simulink model "Model1"  (R2020a)
settings: Solver=VariableStepAuto  StartTime=0.0  StopTime=1600 * SimPars.SampleTime  RelTol=1e-3
undefined symbols (not defined in the file or in its folder): pskmod, SimPars
libraries: commutil2 x4, commdigbbndpm3 x3, dspsigops x2, commsequence2 x2, commsync2 x2, commfilt2 x2, commrflib2 x1, commsink2 x1, commrfcorlib x1, dspstat3 x1, commrandsrc3 x1, dspmathops x1
settings Model: Creator=esha_  LastModifiedBy=esha_

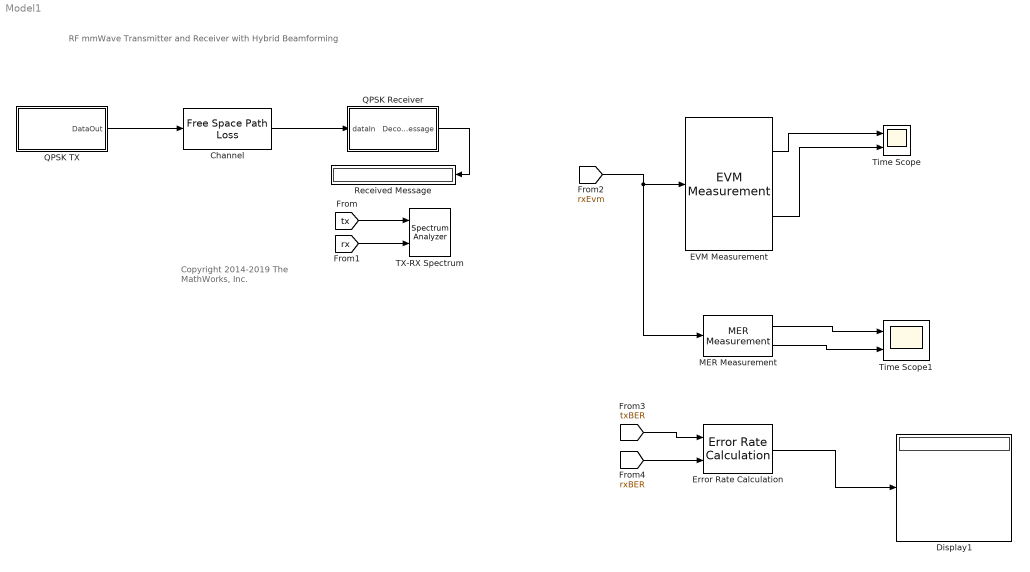
== system Model1 ==
  note: RF mmWave Transmitter and Receiver with Hybrid Beamforming
  note: Copyright 2014-2019 The MathWorks, Inc.
  Channel : commrflib2/Free Space Path Loss  mode=Decibels  dB=5  d=0.100  fc=1920
      settings: SourceProductBaseCode=CM
  Display1 : Display
  EVM Measurement : commutil2/EVM Measurement  Normalization=Average reference signal power  AverageConstellationPower=1  PeakConstellationPower=1  ReferenceSignalSource=Estimated from reference constellation  ReferenceConstellation=pskmod((0:3),4,pi/4)  MeasurementIntervalSource=Input length  MeasurementInterval=100  AveragingDimensions=1  MaximumEVMOutputPort=on  XPercentileEVMOutputPort=off  XPercentileValue=95  SymbolCountOutputPort=on  SimulateUsing=Interpreted execution
      settings: SourceProductBaseCode=CM
  Error Rate Calculation : commsink2/Error Rate Calculation  N=0  st_delay=0  cp_mode=Entire frame  subframe=[]  PMode=Port  WsName=ErrorVec  RsMode2=off  stop=off  numErr=100  maxBits=1e6
  MER Measurement : commutil2/MER Measurement  ReferenceSignalSource=Estimated from reference constellation  ReferenceConstellation=pskmod((0:3),4,pi/4)  MeasurementIntervalSource=Input length  MeasurementInterval=100  AveragingDimensions=1  MinimumMEROutputPort=on  XPercentileMEROutputPort=off  XPercentileValue=95  SymbolCountOutputPort=off  SimulateUsing=Interpreted execution
      settings: SourceProductBaseCode=CM
  QPSK Receiver : Subsystem
      mask Display: disp('QPSK \n Receiver');
  QPSK TX : Subsystem  mask{Power=-10}
      mask prompts: Power "Power (dBFS)"
      mask Display: disp('QPSK \n Transmitter')
  Received Message : Display
  TX-RX Spectrum : SpectrumAnalyzer  NumInputPorts=2
  Time Scope : Scope  NumInputPorts=2
      settings: Description=EVM
  Time Scope1 : Scope  NumInputPorts=2
      settings: Description=SNR
  wires:
  [rx] -> TX-RX Spectrum/2
  QPSK Receiver/1(Decoded Message) -> Received Message/1
  [tx] -> TX-RX Spectrum/1
  QPSK TX/1(DataOut) -> Channel/1
  Channel/1 -> QPSK Receiver/1(dataIn)
  EVM Measurement/1 -> Time Scope/1
  EVM Measurement/2 -> Time Scope/2
  [rxEvm] -> MER Measurement/1, EVM Measurement/1
  MER Measurement/1 -> Time Scope1/1
  MER Measurement/2 -> Time Scope1/2
  Error Rate Calculation/1 -> Display1/1
  [txBER] -> Error Rate Calculation/1
  [rxBER] -> Error Rate Calculation/2

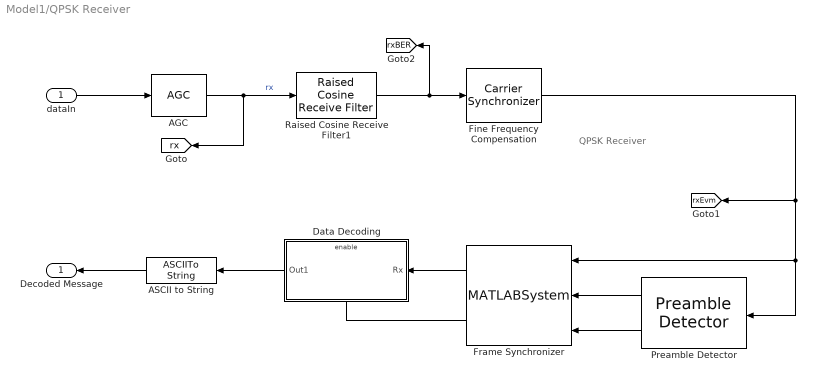
== system Model1/QPSK Receiver ==
  note: QPSK Receiver
  dataIn : Inport
  AGC : commrfcorlib/AGC  LegacyMode=off  DetectorMethod=Rectifier  LoopMethod=Linear  UpdatePeriod=100  StepSize=0.1  AdaptationStepSize=0.01  DesiredOutputPower=1  AveragingLength=200  MaximumGain=30  MaxPowerGain=60  GainOutputPort=off  InputPowerOutputPort=off  SimulateUsing=Code generation
  ASCII to String : ASCIIToString
  Data Decoding : Subsystem
      mask Display: disp('Data Decoding');
  Fine Frequency Compensation : commsync2/Carrier Synchronizer  Modulation=QPSK  ModulationPhaseOffset=Auto  CustomPhaseOffset=0  SamplesPerSymbol=1  DampingFactor=1/sqrt(2)  NormalizedLoopBandwidth=0.005  EstimatedPhaseErrorOutputPort=off  SimulateUsing=Code generation
  Frame Synchronizer : MATLABSystem  System=comm.internal.examples.FrameSynchronizer  Input=Symbol  OutputFrameLength=SimPars.NumSymsPerFrame  PreambleLength=SimPars.BarkerLength  SimulateUsing=Code generation
      mask Type: comm.internal.examples.FrameSynchronizer
      mask Display:
      | disp(['Frame' char(10) 'Synchronizer']);
      | port_label('input',1,'u');
      | port_label('input',2,'idx');
      | port_label('input',3,'dtMt');
      | port_label('output',1,'Frame');
      | port_label('output',2,'Valid');
  Preamble Detector : commsync2/Preamble Detector  Input=Symbol  Preamble=sqrt(2)/2 * (-1-1i) *SimPars.BarkerCode  Threshold=10  DetectionMetricOutput=on  Detections=All  SimulateUsing=Code generation
      settings: SourceProductBaseCode=CM
  Raised Cosine Receive Filter1 : commfilt2/Raised Cosine Receive Filter  filtType=Square root  R=SimPars.RolloffFactor  filtSpan=SimPars.RCFilterSpan  N=SimPars.SamplesPerSymbol  downFactor=SimPars.RxRCFilterDecimation  downOffset=0  filterGain=1  InputProcessing=Columns as channels (frame based)  RateOptions=Enforce single-rate processing  framing=Mute  checkCoeff=off  variableName=rcRxFilt1  currentFiltSpan=10  D=5  inputOffset=0  sampMode=Mute  saveAsFlag=0  rateMode=Downsampling  checkGain=Normalized  launchFVT=on  roundingMode=Floor  overflowMode=off  coeffDataTypeStr=Inherit: Same word length as input  coeffMin=[]  coeffMax=[]  coeffLastDataTypeStr=Inherit: Same word length as input  accumDataTypeStr=Inherit: Same as product output  accumLastDataTypeStr=Inherit: Same as product output  outputDataTypeStr=Inherit: Same as accumulator  outputMin=[]  outputMax=[]  outputLastDataTypeStr=Inherit: Same as accumulator
  Decoded Message : Outport  VectorParamsAs1DForOutWhenUnconnected=off
  tag scope: rx=global, rxBER=global, rxEvm=global
  wires:
  ASCII to String/1 -> Decoded Message/1
  Data Decoding/1(Out1) -> ASCII to String/1
  AGC/1 -> Raised Cosine Receive Filter1/1, [rx]  "rx"
  Preamble Detector/1 -> Frame Synchronizer/2
  Frame Synchronizer/2 -> Data Decoding/Enable
  Frame Synchronizer/1 -> Data Decoding/1(Rx)
  Preamble Detector/2 -> Frame Synchronizer/3
  Fine Frequency Compensation/1 -> [rxEvm], Frame Synchronizer/1, Preamble Detector/1
  dataIn/1 -> AGC/1
  Raised Cosine Receive Filter1/1 -> [rxBER], Fine Frequency Compensation/1

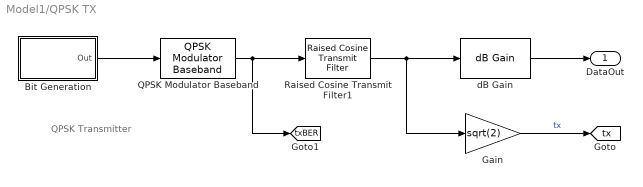
== system Model1/QPSK TX ==
  note: QPSK Transmitter
  Bit Generation : Subsystem
      mask Display: disp('Bits Generation')
  Gain : Gain  Gain=sqrt(2)
  QPSK Modulator Baseband : commdigbbndpm3/QPSK Modulator Baseband  InType=Bit  Enc=Gray  Ph=pi/4  outDtype=double  outWordLen=16  outUDDataType=sfix(16)  outFracLenMode=Best precision  outFracLen=15  outDataTypeStr=double  outLastDataTypeStr=double
  Raised Cosine Transmit Filter1 : commfilt2/Raised Cosine Transmit Filter  filtType=Square root  R=SimPars.RolloffFactor  filtSpan=SimPars.RCFilterSpan  N=SimPars.SamplesPerSymbol  filterGain=1  InputProcessing=Columns as channels (frame based)  RateOptions=Enforce single-rate processing  framing=Mute  checkCoeff=off  variableName=rcTxFilt1  checkGain=Normalized  sampMode=Mute  saveAsFlag=0  currentFiltSpan=10  D=5  launchFVT=on  roundingMode=Floor  overflowMode=off  coeffDataTypeStr=Inherit: Same word length as input  coeffMin=[]  coeffMax=[]  coeffLastDataTypeStr=Inherit: Same word length as input  outputDataTypeStr=Inherit: Same as accumulator  outputMin=[]  outputMax=[]  outputLastDataTypeStr=Inherit: Same as accumulator
  dB Gain : dspmathops/dB Gain  dB=Power-30+3  intype=Amplitude
      settings: SourceProductBaseCode=DS
  DataOut : Outport  VectorParamsAs1DForOutWhenUnconnected=off
  tag scope: tx=global, txBER=global
  wires:
  dB Gain/1 -> DataOut/1
  Bit Generation/1(Out) -> QPSK Modulator Baseband/1
  QPSK Modulator Baseband/1 -> [txBER], Raised Cosine Transmit Filter1/1
  Raised Cosine Transmit Filter1/1 -> Gain/1, dB Gain/1
  Gain/1 -> [tx]  "tx"

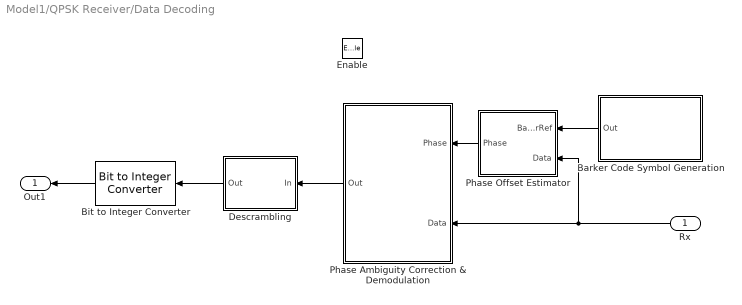
== system Model1/QPSK Receiver/Data Decoding ==
  Rx : Inport
  Enable : EnablePort
  "Barker Code Symbol Generation " : Subsystem
      mask Display: disp('Barker Code\nSymbol Generation')
  Bit to Integer Converter : commutil2/Bit to Integer Converter  nbits=7  bitOrder=MSB first  signedOutputValues=Unsigned  outDtype=Inherit via internal rule  outDtypeSigned=Inherit via internal rule
  Descrambling : Subsystem
      mask Display: disp('Descrambling');
  Phase Ambiguity Correction & Demodulation : Subsystem
      mask Display: disp('Phase Ambiguity\nCorrection\n& Demodulation');
  Phase Offset Estimator : Subsystem
  Out1 : Outport  VectorParamsAs1DForOutWhenUnconnected=off
  wires:
  "Barker Code Symbol Generation "/1(Out) -> Phase Offset Estimator/1(BarkerRef)
  Phase Offset Estimator/1(Phase) -> Phase Ambiguity Correction & Demodulation/1(Phase)
  Rx/1 -> Phase Offset Estimator/2(Data), Phase Ambiguity Correction & Demodulation/2(Data)
  Descrambling/1(Out) -> Bit to Integer Converter/1
  Phase Ambiguity Correction & Demodulation/1(Out) -> Descrambling/1(In)
  Bit to Integer Converter/1 -> Out1/1

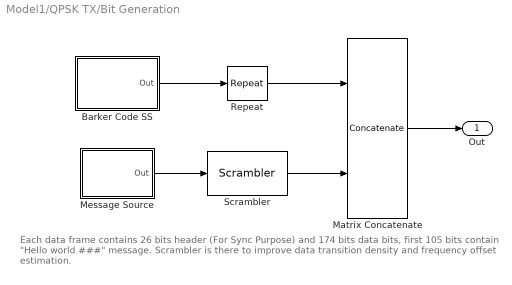
== system Model1/QPSK TX/Bit Generation ==
  note: Each data frame contains 26 bits header (For Sync Purpose) and 174 bits data bits, first 105 bits contain "Hello world ###" message. Scrambler is there to improve data transition density and frequency offset estimation.
  Barker Code SS : Subsystem
      mask Display: disp('Unipolar\nBarker Code')
  Matrix Concatenate : Concatenate  Mode=Multidimensional array
  Message Source : Subsystem
      mask Display: disp('Message\nSource')
  Repeat : dspsigops/Repeat  N=2  InputProcessing=Columns as channels (frame based)  RateOptions=Enforce single-rate processing  ic=0  mode=Unused parameter value
  Scrambler : commsequence2/Scrambler  M=2  poly=[1 1 1 0 1]  iniStaSource=Dialog Parameter  ini_sta=[0 0 0 0]  resetViaPort=off
      settings: SourceProductBaseCode=CM
  Out : Outport  VectorParamsAs1DForOutWhenUnconnected=off
  wires:
  Barker Code SS/1(Out) -> Repeat/1
  Matrix Concatenate/1 -> Out/1
  Message Source/1(Out) -> Scrambler/1
  Repeat/1 -> Matrix Concatenate/1
  Scrambler/1 -> Matrix Concatenate/2

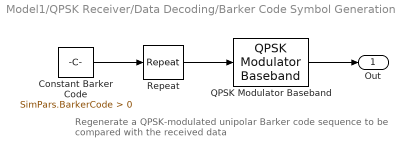
== system Model1/QPSK Receiver/Data Decoding/Barker Code Symbol Generation  ==
  note: Regenerate a QPSK-modulated unipolar Barker code sequence
      | to be compared with the received data
  Constant Barker Code : Constant  Value=SimPars.BarkerCode > 0  VectorParams1D=off  OutDataTypeStr=double
  QPSK Modulator Baseband : commdigbbndpm3/QPSK Modulator Baseband  InType=Bit  Enc=Gray  Ph=pi/4  outDtype=double  outWordLen=16  outUDDataType=sfix(16)  outFracLenMode=Best precision  outFracLen=15  outDataTypeStr=double  outLastDataTypeStr=double
  Repeat : dspsigops/Repeat  N=2  InputProcessing=Columns as channels (frame based)  RateOptions=Enforce single-rate processing  ic=0  mode=Unused parameter value
  Out : Outport  VectorParamsAs1DForOutWhenUnconnected=off
  wires:
  Constant Barker Code/1 -> Repeat/1
  Repeat/1 -> QPSK Modulator Baseband/1
  QPSK Modulator Baseband/1 -> Out/1

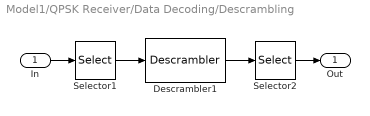
== system Model1/QPSK Receiver/Data Decoding/Descrambling ==
  In : Inport
  Descrambler1 : commsequence2/Descrambler  M=2  poly=[1 1 1 0 1]  iniStaSource=Dialog Parameter  ini_sta=[0 0 0 0]  resetViaPort=off
      settings: SourceProductBaseCode=CM
  Selector1 : Selector  IndexOptions=Index vector (dialog)  Indices=[2*SimPars.BarkerLength+1:SimPars.NumBitsPerFrame]  OutputSizes=1
  Selector2 : Selector  IndexOptions=Index vector (dialog)  Indices=[1:SimPars.NumMsgBits]  OutputSizes=1
  Out : Outport  VectorParamsAs1DForOutWhenUnconnected=off
  wires:
  In/1 -> Selector1/1
  Selector1/1 -> Descrambler1/1
  Descrambler1/1 -> Selector2/1
  Selector2/1 -> Out/1

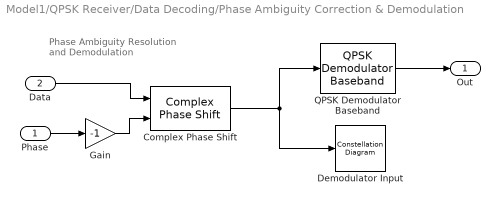
== system Model1/QPSK Receiver/Data Decoding/Phase Ambiguity Correction & Demodulation ==
  note: Phase Ambiguity Resolution
      | and Demodulation
  Phase : Inport
  Data : Inport  Port=2
  Complex Phase Shift : commutil2/Complex Phase Shift
      settings: SourceProductBaseCode=CM
  Demodulator Input : ConstellationDiagram
  Gain : Gain  Gain=-1  OutDataTypeStr=Inherit: Same as input
  QPSK Demodulator Baseband : commdigbbndpm3/QPSK Demodulator Baseband  OutType=Bit  DecType=Hard decision  VarSource=Dialog  Variance=1  Dec=Gray  Ph=pi/4  outDtype1=Inherit via internal rule  outDtype2=Inherit via internal rule  derotateFactorWordLen=16  derotateFactorDataTypeStr=Inherit: Same word length as input  derotateFactorLastDataTypeStr=Inherit: Same word length as input
  Out : Outport  VectorParamsAs1DForOutWhenUnconnected=off
  wires:
  Phase/1 -> Gain/1
  Complex Phase Shift/1 -> Demodulator Input/1, QPSK Demodulator Baseband/1
  QPSK Demodulator Baseband/1 -> Out/1
  Gain/1 -> Complex Phase Shift/2
  Data/1 -> Complex Phase Shift/1

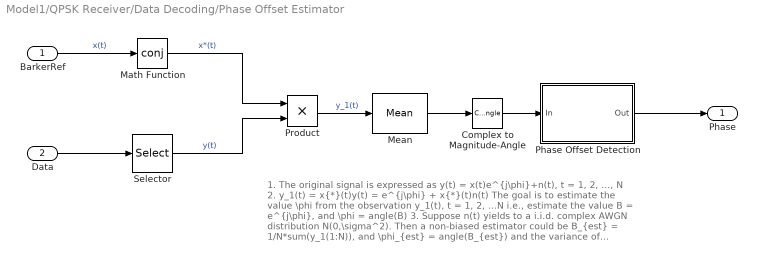
== system Model1/QPSK Receiver/Data Decoding/Phase Offset Estimator ==
  note: 1. The original signal is expressed as y(t) = x(t)e^{j\phi}+n(t), t = 1, 2, ..., N
      | 2. y_1(t) = x{*}(t)y(t) = e^{j\phi} + x{*}(t)n(t)
      | The goal is to estimate the value \phi from the observation y_1(t), t = 1, 2, ...N
      | i.e., estimate the value B = e^{j\phi}, and \phi = angle(B)
      | 3. Suppose n(t) yields to a i.i.d. complex AWGN distribution N(0,\sigma^2).
      | Then a non-biased estimator could be
      | B_{est} = 1/N*sum(y_1(1:N)), and \phi_{est} = angle(B_{est})
      | and the variance of B_{est} is \sigma^2/N
  BarkerRef : Inport
  Data : Inport  Port=2
  Complex to Magnitude-Angle : ComplexToMagnitudeAngle  Output=Angle
  Math Function : Math  Operator=conj  SignedPower=on  SaturateOnIntegerOverflow=on
  Mean : dspstat3/Mean  run=off  InputProcessing=Columns as channels (frame based)  reset_popup=None  directionMode=Each column  dimension=1  roiEnable=off  roiType=Rectangles  roiPortion=Entire ROI  roiOutput=Individual statistics for each ROI  roiFlag=off  roundingMode=Floor  overflowMode=off  outputDataTypeStr=Inherit: Same as accumulator  outputMin=[]  outputMax=[]  outputLastDataTypeStr=Inherit: Same as accumulator
  Phase Offset Detection : MATLAB Function  TreatAsAtomicUnit=on
  Product : Product  RndMeth=Zero
  Selector : Selector  IndexOptions=Index vector (dialog)  Indices=[1:SimPars.BarkerLength]  OutputSizes=1
  Phase : Outport  VectorParamsAs1DForOutWhenUnconnected=off
  wires:
  Data/1 -> Selector/1
  BarkerRef/1 -> Math Function/1  "x(t)"
  Selector/1 -> Product/2  "y(t)"
  Math Function/1 -> Product/1  "x*(t)"
  Product/1 -> Mean/1  "y_1(t)"
  Mean/1 -> Complex to Magnitude-Angle/1
  Complex to Magnitude-Angle/1 -> Phase Offset Detection/1(In)
  Phase Offset Detection/1(Out) -> Phase/1

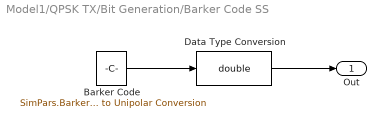
== system Model1/QPSK TX/Bit Generation/Barker Code SS ==
  Barker Code : Constant  Value="SimPars.BarkerCode > 0  % Bipolar to Unipolar Conversion"  VectorParams1D=off
  Data Type Conversion : DataTypeConversion  OutDataTypeStr=double
  Out : Outport  VectorParamsAs1DForOutWhenUnconnected=off
  wires:
  Barker Code/1 -> Data Type Conversion/1
  Data Type Conversion/1 -> Out/1

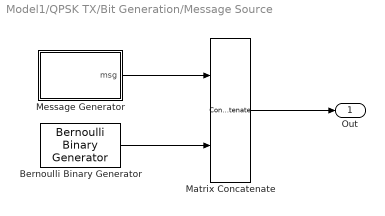
== system Model1/QPSK TX/Bit Generation/Message Source ==
  Bernoulli Binary Generator : commrandsrc3/Bernoulli Binary Generator  ProbabilityOfZero=0.5  SeedSource=Parameter  Seed=61  SampleTime=SimPars.BernoulliSampleTime  SamplesPerFrame=SimPars.BernoulliFrameBits  OutputDataType=double  SimulateUsing=Code generation
  Matrix Concatenate : Concatenate  Mode=Multidimensional array
  Message Generator : MATLAB Function  TreatAsAtomicUnit=on
  Out : Outport  VectorParamsAs1DForOutWhenUnconnected=off
  wires:
  Message Generator/1(msg) -> Matrix Concatenate/1
  Bernoulli Binary Generator/1 -> Matrix Concatenate/2
  Matrix Concatenate/1 -> Out/1

== matlab function Model1/QPSK TX/Bit Generation/Message Source/Message Generator ==
  data: msg output
function msg = genMsg
%#codegen
persistent msgStrSet count;
if isempty(msgStrSet)
    count = 0;
    msgStrSet = [
        'Hello world 000';                                              ...
        'Hello world 001';                                              ...
        'Hello world 002';                                              ...
        'Hello world 003';                                              ...
        'Hello world 004';                                              ...
        'Hello world 005';                                              ...
        'Hello world 006';                                              ...
        'Hello world 007';                                              ...
        'Hello world 008';                                              ...
        'Hello world 009';                                              ...
        'Hello world 010';                                              ...
        'Hello world 011';                                              ...
        'Hello world 012';                                              ...
        'Hello world 013';                                              ...
        'Hello world 014';                                              ...
        'Hello world 015';                                              ...
        'Hello world 016';                                              ...
        'Hello world 017';                                              ...
        'Hello world 018';                                              ...
        'Hello world 019';                                              ...
        'Hello world 020';                                              ...
        'Hello world 021';                                              ...
        'Hello world 022';                                              ...
        'Hello world 023';                                              ...
        'Hello world 024';                                              ...
        'Hello world 025';                                              ...
        'Hello world 026';                                              ...
        'Hello world 027';                                              ...
        'Hello world 028';                                              ...
        'Hello world 029';                                              ...
        'Hello world 030';                                              ...
        'Hello world 031';                                              ...
        'Hello world 032';                                              ...
        'Hello world 033';                                              ...
        'Hello world 034';                                              ...
        'Hello world 035';                                              ...
        'Hello world 036';                                              ...
        'Hello world 037';                                              ...
        'Hello world 038';                                              ...
        'Hello world 039';                                              ...
        'Hello world 040';                                              ...
        'Hello world 041';                                              ...
        'Hello world 042';                                              ...
        'Hello world 043';                                              ...
        'Hello world 044';                                              ...
        'Hello world 045';                                              ...
        'Hello world 046';                                              ...
        'Hello world 047';                                              ...
        'Hello world 048';                                              ...
        'Hello world 049';                                              ...
        'Hello world 050';                                              ...
        'Hello world 051';                                              ...
        'Hello world 052';                                              ...
        'Hello world 053';                                              ...
        'Hello world 054';                                              ...
        'Hello world 055';                                              ...
        'Hello world 056';                                              ...
        'Hello world 057';                                              ...
        'Hello world 058';                                              ...
        'Hello world 059';                                              ...
        'Hello world 060';                                              ...
        'Hello world 061';                                              ...
        'Hello world 062';                                              ...
        'Hello world 063';                                              ...
        'Hello world 064';                                              ...
        'Hello world 065';                                              ...
        'Hello world 066';                                              ...
        'Hello world 067';                                              ...
        'Hello world 068';                                              ...
        'Hello world 069';                                              ...
        'Hello world 070';                                              ...
        'Hello world 071';                                              ...
        'Hello world 072';                                              ...
        'Hello world 073';                                              ...
        'Hello world 074';                                              ...
        'Hello world 075';                                              ...
        'Hello world 076';                                              ...
        'Hello world 077';                                              ...
        'Hello world 078';                                              ...
        'Hello world 079';                                              ...
        'Hello world 080';                                              ...
        'Hello world 081';                                              ...
        'Hello world 082';                                              ...
        'Hello world 083';                                              ...
        'Hello world 084';                                              ...
        'Hello world 085';                                              ...
        'Hello world 086';                                              ...
        'Hello world 087';                                              ...
        'Hello world 088';                                              ...
        'Hello world 089';                                              ...
        'Hello world 090';                                              ...
        'Hello world 091';                                              ...
        'Hello world 092';                                              ...
        'Hello world 093';                                              ...
        'Hello world 094';                                              ...
        'Hello world 095';                                              ...
        'Hello world 096';                                              ...
        'Hello world 097';                                              ...
        'Hello world 098';                                              ...
        'Hello world 099'];
end

msgStr = msgStrSet(count+1,:);
msgBin = de2bi(int8(msgStr),7,'left-msb');
msg = reshape(double(msgBin).',105,1);
count = mod(count+1,100);

== matlab function Model1/QPSK Receiver/Data Decoding/Phase Offset Estimator/Phase Offset Detection ==
  data: In input; Out output
function Out = phasedecision(In)
% Map the estimated phase to one of -pi, -pi/2, 0, pi/2,  
%#codegen
Out = round(In.*2./pi)./2.*pi;
% The above processing is equivalent to the following processing using
% if/else statements
%
% if In<pi/4 && In>-pi/4
%     Out = 0;
% elseif In>=pi/4 && In<pi*3/4
%     Out = pi/2;
% elseif In>=pi*3/4 || In<=-pi*3/4
%     Out = -pi;
% else
%     Out = -pi/2;
% end
